simulink model "BMS_ClosedLoop"  (R2019b)
settings: configuration reference "BMS_Sw_CodeGenConfig" (kept outside this file)
values from neighbouring files (symbols this model uses):
  Ns_Module = 6.0    [Battery_16Packs_1RC.sldd]
  NumModules = 16.0    [Battery_16Packs_1RC.sldd]
CloseFcn:
  | cleanDictionaries
settings Model: DataDictionary=Battery_System_DD.sldd  EnableAccessToBaseWorkspace=off  PauseTimes=0  OrderedModelArguments=off  Creator=mluethy  LastModifiedBy=ZHOU Jinhan
settings ConfigSetRef: SourceName=BMS_Sw_CodeGenConfig

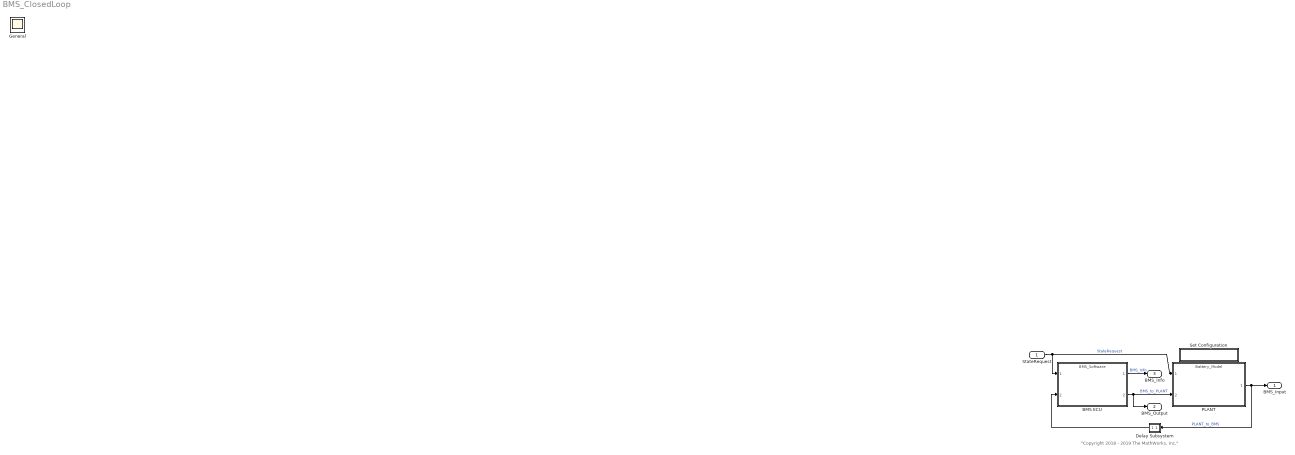
== system BMS_ClosedLoop ==
  note: "Copyright 2018 - 2019 The MathWorks, Inc."
  StateRequest : Inport  OutDataTypeStr=Enum: SRE
  BMS ECU : ModelReference  ModelNameDialog=BMS_Software  SimulationMode=Normal  ModelReferenceVersion=1.696
      mask Display: image('Microcontroller.jpg',[50,17,58,48])
  Delay Subsystem : Subsystem
      mask Display: image('Delay.JPG');
  PLANT : ModelReference  ModelNameDialog=Battery_Model  ModelReferenceVersion=1.555
      mask Display: image('Plant_Battery.jpg',[40,15,80,48])
  Set Configuration : Subsystem
      mask Display: disp('Set Plant Configuration');
  BMS_Input : Outport  OutDataTypeStr=Bus: BMS_Input  VectorParamsAs1DForOutWhenUnconnected=off
  BMS_Output : Outport  Port=2  OutDataTypeStr=Bus: BMS_Output  VectorParamsAs1DForOutWhenUnconnected=off
  BMS_Info : Outport  Port=3  OutDataTypeStr=Bus: BMS_Info  VectorParamsAs1DForOutWhenUnconnected=off  BusOutputAsStruct=on
  General : Scope
  wires:
  StateRequest/1 -> PLANT/1, BMS ECU/1  "StateRequest"
  PLANT/1 -> Delay Subsystem/1(FROM_PLANT), BMS_Input/1  "PLANT_to_BMS"
  BMS ECU/1 -> BMS_Info/1  "BMS_Info"
  BMS ECU/2 -> PLANT/2, BMS_Output/1  "BMS_to_PLANT"
  Delay Subsystem/1(OutBus) -> BMS ECU/2

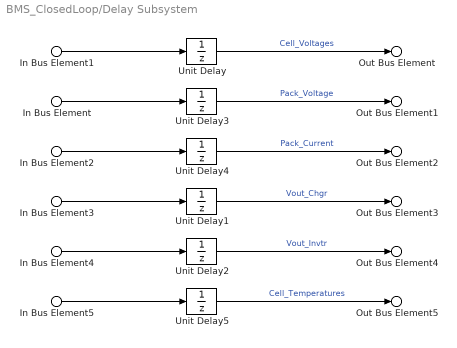
== system BMS_ClosedLoop/Delay Subsystem ==
  In Bus Element1 : Inport  PortName=FROM_PLANT  Element=Cell_Voltages
  In Bus Element : Inport  PortName=FROM_PLANT  Element=Pack_Voltage
  In Bus Element2 : Inport  PortName=FROM_PLANT  Element=Pack_Current
  In Bus Element3 : Inport  PortName=FROM_PLANT  Element=Vout_Chgr
  In Bus Element4 : Inport  PortName=FROM_PLANT  Element=Vout_Invtr
  In Bus Element5 : Inport  PortName=FROM_PLANT  Element=Cell_Temperatures
  Unit Delay : UnitDelay  InitialCondition=3.6*ones(1, Ns_Module*NumModules)  SampleTime=-1  HasFrameUpgradeWarning=on
  Unit Delay1 : UnitDelay  SampleTime=-1  HasFrameUpgradeWarning=on
  Unit Delay2 : UnitDelay  SampleTime=-1  HasFrameUpgradeWarning=on
  Unit Delay3 : UnitDelay  InitialCondition=3.6*Ns_Module*NumModules  SampleTime=-1  HasFrameUpgradeWarning=on
  Unit Delay4 : UnitDelay  SampleTime=-1  HasFrameUpgradeWarning=on
  Unit Delay5 : UnitDelay  InitialCondition=293.15*ones(1,Ns_Module*NumModules)  SampleTime=-1  HasFrameUpgradeWarning=on
  Out Bus Element : Outport  VectorParamsAs1DForOutWhenUnconnected=off  PortName=OutBus  Element=Cell_Voltages
  Out Bus Element1 : Outport  VectorParamsAs1DForOutWhenUnconnected=off  PortName=OutBus  Element=Pack_Voltage
  Out Bus Element2 : Outport  VectorParamsAs1DForOutWhenUnconnected=off  PortName=OutBus  Element=Pack_Current
  Out Bus Element3 : Outport  VectorParamsAs1DForOutWhenUnconnected=off  PortName=OutBus  Element=Vout_Chgr
  Out Bus Element4 : Outport  VectorParamsAs1DForOutWhenUnconnected=off  PortName=OutBus  Element=Vout_Invtr
  Out Bus Element5 : Outport  VectorParamsAs1DForOutWhenUnconnected=off  PortName=OutBus  Element=Cell_Temperatures
  wires:
  Unit Delay1/1 -> Out Bus Element3/1  "Vout_Chgr"
  Unit Delay2/1 -> Out Bus Element4/1  "Vout_Invtr"
  Unit Delay5/1 -> Out Bus Element5/1  "Cell_Temperatures"
  Unit Delay4/1 -> Out Bus Element2/1  "Pack_Current"
  Unit Delay/1 -> Out Bus Element/1  "Cell_Voltages"
  Unit Delay3/1 -> Out Bus Element1/1  "Pack_Voltage"
  In Bus Element1/1 -> Unit Delay/1
  In Bus Element/1 -> Unit Delay3/1
  In Bus Element2/1 -> Unit Delay4/1
  In Bus Element3/1 -> Unit Delay1/1
  In Bus Element4/1 -> Unit Delay2/1
  In Bus Element5/1 -> Unit Delay5/1

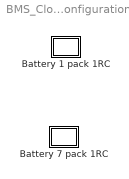
== system BMS_ClosedLoop/Set Configuration ==
  Battery 1 pack 1RC : Subsystem
      settings: OpenFcn=|
      | SharedDictionaryObj = Simulink.data.dictionary.open('Shared_DD.sldd');
      | try removeDataSource(SharedDictionaryObj,'Battery_1Pack_1RC.sldd')
      | end
      | try removeDataSource(SharedDictionaryObj,'Battery_16Packs_1RC.sldd')
      | end
      | addDataSource(SharedDictionaryObj,'Battery_1Pack_1RC.sldd')
  Battery 7 pack 1RC : Subsystem
      settings: OpenFcn=|
      | SharedDictionaryObj = Simulink.data.dictionary.open('Shared_DD.sldd');
      | try removeDataSource(SharedDictionaryObj,'Battery_1Pack_1RC.sldd')
      | end
      | try removeDataSource(SharedDictionaryObj,'Battery_16Packs_1RC.sldd')
      | end
      | addDataSource(SharedDictionaryObj,'Battery_16Packs_1RC.sldd')

== system BMS_ClosedLoop/Set Configuration/Battery 1 pack 1RC ==

== system BMS_ClosedLoop/Set Configuration/Battery 7 pack 1RC ==
